simulink model "InjectorTiming"  (R2021a)
settings: Solver=FixedStepDiscrete  StartTime=0.0  StopTime=10.0  FixedStep=0.15  RelTol=1e-3
settings Model: Creator=A  LastModifiedBy=mulla

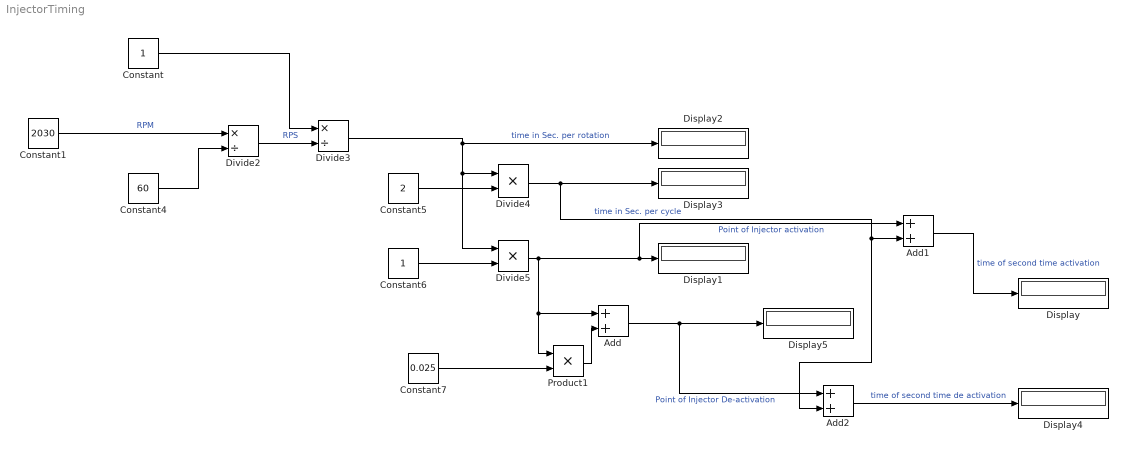
== system InjectorTiming ==
  Add : Sum
  Add1 : Sum
  Add2 : Sum
  Constant : Constant
  Constant1 : Constant  Value=2030
  Constant4 : Constant  Value=60
  Constant5 : Constant  Value=2
  Constant6 : Constant
  Constant7 : Constant  Value=0.025
  Display{,1..5} (6 alike) : Display
  Divide2 : Product  Inputs=*/
  Divide3 : Product  Inputs=*/
  Divide4 : Product  Inputs=**
  Divide5 : Product  Inputs=**
  Product1 : Product
  wires:
  Divide3/1 -> Display2/1, Divide5/1, Divide4/1  "time in Sec. per rotation"
  Constant6/1 -> Divide5/2
  Divide4/1 -> Add2/2, Add1/2, Display3/1  "time in Sec. per cycle"
  Constant4/1 -> Divide2/2
  Constant5/1 -> Divide4/2
  Product1/1 -> Add/2
  Divide2/1 -> Divide3/2  "RPS"
  Divide5/1 -> Add1/1, Display1/1, Add/1, Product1/1  "Point of Injector activation"
  Add/1 -> Add2/1, Display5/1  "Point of Injector De-activation"
  Constant7/1 -> Product1/2
  Constant1/1 -> Divide2/1  "RPM"
  Constant/1 -> Divide3/1
  Add2/1 -> Display4/1  "time of second time de activation"
  Add1/1 -> Display/1  "time of second time activation"
